simulink model "drone_nao_linear_V3"  (R2015a)
settings: Solver=ode45  StartTime=0.0  StopTime=14  RelTol=1e-3
values from neighbouring files (symbols this model uses):
  Cx = 0.3    [dados_ar_drone.m]
  Cy = 0.1    [dados_ar_drone.m]
  d_fi = 0.5    [dados_ar_drone.m]
  d_teta = 0.5    [dados_ar_drone.m]
  Fi_max = 0.26    [dados_ar_drone.m]
  g = 9.8    [dados_ar_drone.m]
  K_psi_p = 1    [dados_ar_drone.m]
  K_z_p = 1.3    [dados_ar_drone.m]
  omega_fi = 4.47    [dados_ar_drone.m]
  omega_teta = 4.47    [dados_ar_drone.m]
  Psi_p_max = 1.74    [dados_ar_drone.m]
  T = 7.5    [dados_ar_drone.m]
  Tau_psi_p = 0.3    [dados_ar_drone.m]
  Tau_z_p = 0.4    [dados_ar_drone.m]
  Teta_max = 0.26    [dados_ar_drone.m]
  z_p_max = 1    [dados_ar_drone.m]
libraries: simulink_extras x5
settings Model: Creator=Humberto  LastModifiedBy=Humberto

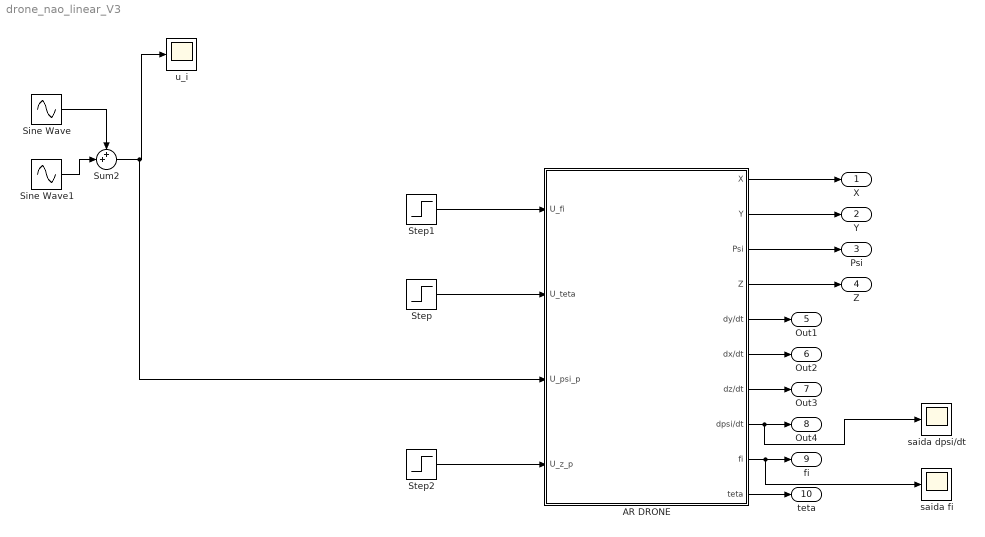
== system drone_nao_linear_V3 ==
  AR DRONE : Subsystem
      mask Display:
      | color('blue');port_label('output',1,'x')
      | image('ardrone2.0')
  Sine Wave : Sin  Amplitude=0.5  Frequency=2*pi/T  SampleTime=0
  Sine Wave1 : Sin  Amplitude=0.3  Frequency=2*pi/(0.2*T)  SampleTime=0
  Step : Step  Time=0  After=0  SampleTime=0
  Step1 : Step  Time=0  After=0  SampleTime=0
  Step2 : Step  Time=0  After=0  SampleTime=0
  Sum2 : Sum  Inputs=++|
  saida dpsi/dt : Scope
      settings: SaveName=ScopeData13
  saida fi : Scope
      settings: SaveName=ScopeData10
  u_i : Scope
      settings: SaveName=ScopeData8
  X : Outport
  Y : Outport  Port=2
  Psi : Outport  Port=3
  Z : Outport  Port=4
  Out1 : Outport  Port=5
  Out2 : Outport  Port=6
  Out3 : Outport  Port=7
  Out4 : Outport  Port=8
  fi : Outport  Port=9
  teta : Outport  Port=10
  wires:
  Sine Wave/1 -> Sum2/1
  Sine Wave1/1 -> Sum2/2
  Sum2/1 -> AR DRONE/3(U_psi_p), u_i/1
  Step/1 -> AR DRONE/2(U_teta)
  Step2/1 -> AR DRONE/4(U_z_p)
  AR DRONE/2(Y) -> Y/1
  AR DRONE/3(Psi) -> Psi/1
  AR DRONE/4(Z) -> Z/1
  AR DRONE/1(X) -> X/1
  AR DRONE/10(teta) -> teta/1
  AR DRONE/5(dy/dt) -> Out1/1
  AR DRONE/6(dx/dt) -> Out2/1
  AR DRONE/7(dz/dt) -> Out3/1
  AR DRONE/8(dpsi/dt) -> saida dpsi/dt/1, Out4/1
  AR DRONE/9(fi) -> saida fi/1, fi/1
  Step1/1 -> AR DRONE/1(U_fi)

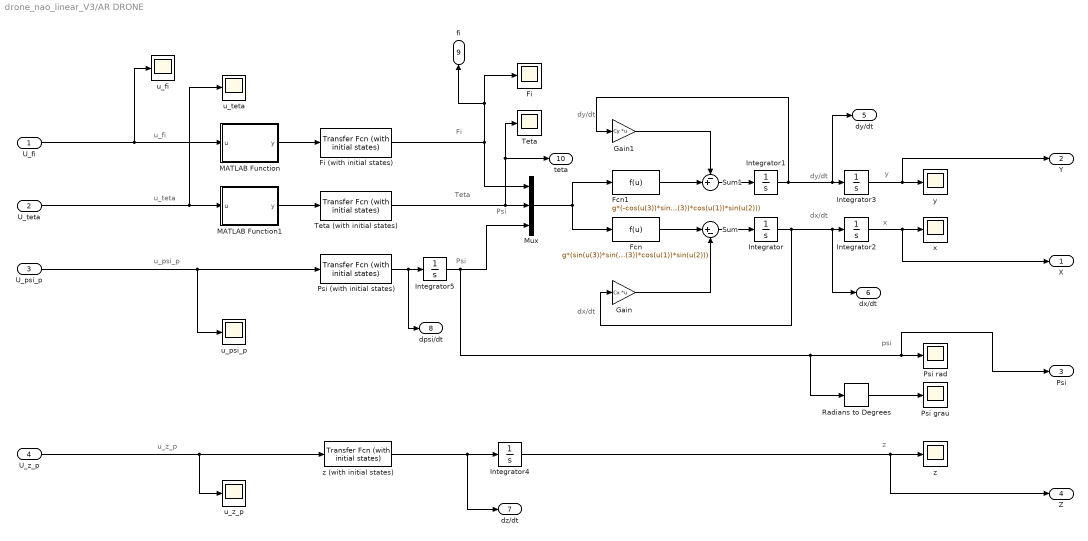
== system drone_nao_linear_V3/AR DRONE ==
  note: z
  note: psi
  note: Psi
  note: Teta
  note: Fi
  note: u_fi
  note: Psi
  note: y
  note: dx/dt
  note: dy/dt
  note: x
  note: dx/dt
  note: dy/dt
  note: u_teta
  note: u_psi_p
  note: u_z_p
  U_fi : Inport
  U_teta : Inport  Port=2
  U_psi_p : Inport  Port=3
  U_z_p : Inport  Port=4
  Fcn : Fcn  Expr=g*(sin(u(3))*sin(u(1))+cos(u(3))*cos(u(1))*sin(u(2)))
  Fcn1 : Fcn  Expr=g*(-cos(u(3))*sin(u(1))+sin(u(3))*cos(u(1))*sin(u(2)))
  Fi : Scope
      settings: SaveName=ScopeData5
  Fi (with initial states) : simulink_extras/Additional Linear/Transfer Fcn (with initial states)  N=Fi_max*(omega_fi^2)  D="[1 2*d_fi*omega_fi  omega_fi^2]"  X0=[0 0]
  Gain : Gain  Gain=Cx  Multiplication=Matrix(K*u)
  Gain1 : Gain  Gain=Cy  Multiplication=Matrix(K*u)
  Integrator{,1..5} (6 alike) : Integrator
  MATLAB Function : MATLAB Function  TreatAsAtomicUnit=on
  MATLAB Function1 : MATLAB Function  TreatAsAtomicUnit=on
  Mux : Mux  Inputs=3
  Psi (with initial states) : simulink_extras/Additional Linear/Transfer Fcn (with initial states)  N=K_psi_p*Psi_p_max  D=[Tau_psi_p 1]  X0=[0]
  Psi grau : Scope
      settings: SaveName=ScopeData4
  Psi rad : Scope
      settings: SaveName=ScopeData2
  Radians to Degrees : simulink_extras/Transformations/Radians to Degrees
  Sum : Sum  Inputs=|+-
  Sum1 : Sum  Inputs=-+|
  Teta : Scope
      settings: SaveName=ScopeData7
  Teta (with initial states) : simulink_extras/Additional Linear/Transfer Fcn (with initial states)  N=Teta_max*(omega_teta^2)  D="[1 2*d_teta*omega_teta  omega_teta^2]"  X0=[0 0]
  u_fi : Scope
      settings: SaveName=ScopeData6
  u_psi_p : Scope
      settings: SaveName=ScopeData11
  u_teta : Scope
      settings: SaveName=ScopeData9
  u_z_p : Scope
      settings: SaveName=ScopeData12
  x : Scope
  y : Scope
  z : Scope
      settings: SaveName=ScopeData3
  z (with initial states) : simulink_extras/Additional Linear/Transfer Fcn (with initial states)  N=K_z_p*z_p_max  D=[Tau_z_p 1]  X0=[0]
  X : Outport
  Y : Outport  Port=2
  Psi : Outport  Port=3
  Z : Outport  Port=4
  dy/dt : Outport  Port=5
  dx/dt : Outport  Port=6
  dz/dt : Outport  Port=7
  dpsi/dt : Outport  Port=8
  fi : Outport  Port=9
  teta : Outport  Port=10
  wires:
  Integrator1/1 -> dy/dt/1, Integrator3/1, Gain1/1
  Sum/1 -> Integrator/1
  Fcn/1 -> Sum/1
  Integrator/1 -> dx/dt/1, Integrator2/1, Gain/1
  Gain/1 -> Sum/2
  z (with initial states)/1 -> dz/dt/1, Integrator4/1
  Radians to Degrees/1 -> Psi grau/1
  U_z_p/1 -> z (with initial states)/1, u_z_p/1
  U_fi/1 -> u_fi/1, MATLAB Function/1(u)
  Psi (with initial states)/1 -> dpsi/dt/1, Integrator5/1
  U_psi_p/1 -> u_psi_p/1, Psi (with initial states)/1
  U_teta/1 -> u_teta/1, MATLAB Function1/1(u)
  Gain1/1 -> Sum1/1
  Sum1/1 -> Integrator1/1
  Fcn1/1 -> Sum1/2
  Fi (with initial states)/1 -> Mux/1, fi/1, Fi/1
  MATLAB Function/1(y) -> Fi (with initial states)/1
  MATLAB Function1/1(y) -> Teta (with initial states)/1
  Integrator2/1 -> x/1, X/1
  Integrator3/1 -> Y/1, y/1
  Mux/1 -> Fcn1/1, Fcn/1
  Teta (with initial states)/1 -> teta/1, Teta/1, Mux/2
  Integrator4/1 -> Z/1, z/1
  Integrator5/1 -> Radians to Degrees/1, Psi/1, Psi rad/1, Mux/3

== matlab function drone_nao_linear_V3/AR DRONE/MATLAB Function1 ==
  data: u input; y output
function y = myfcn2(u)

K_teta_min = 1;
K_teta_max = 2;

if abs(u)>=0.5
    u=K_teta_min*u;
else
    u=K_teta_max*u;
end

y = u;

== matlab function drone_nao_linear_V3/AR DRONE/MATLAB Function ==
  data: u input; y output
function y = myfcn1(u)
K_fi_min = 1;
K_fi_max = 2;
if abs(u)>=0.5
    u=K_fi_min*u;
else
    u=K_fi_max*u;
end

y = u;
